simulink model "DFADAS2_SenFus_v1_201204RC_training_210115"  (R2018b)
settings: Solver=FixedStepDiscrete  StartTime=0.0  StopTime=inf  FixedStep=0.002  RelTol=1e-3  EnableMultiTasking=on
PreLoadFcn:
  | RTWConfigurationCB('preloadfcn', bdroot);
libraries: canmsglib x108, simulink x48, canfdmsglib x12
(part 7 of 28)

== system DFADAS2_SenFus_v1_201204RC_training_210115/Signal Input (Input)/Signal Input (10ms) (Input10)/VehInfo/EPS Signal Receive and Processing (EPSRx) ==
  note: Level: 3
  Bus Creator : BusCreator  Inputs=4
  CAN Unpack : canmsglib/CAN Unpack  CANdbFile=F:\LD\3_simulinkModel_13b\TJAHWA\ADAS_D53_PSA1CAN_LiPiao_DLC.dbc  MsgList=EPS_495_PSA1  MsgName=EPS_495_PSA1  MsgIDType=Standard (11-bit identifier)  MsgIdentifier=1173  MsgLength=4  SignalInfo=Power_steering_status$14$2$2$2$1$0$1$0$-Inf$Inf$#State_indicating_steering_or_not$17$1$2$2$1$0$1$0$-Inf$Inf$#State_of_EPS_for_LKA_function$18$3$2$2$1$0$1$0$-Inf$Inf$#Steering_wheel_torque$0$8$2$1$1$0$2.500000e-01$0$-32$3.150000e+01$#Torque_limitation_if_DAE_limit$16$1$2$2$1$0$1$0$-Inf$Inf$#  NSignals=5  IDPort=off  TimestampPort=off  ErrorPort=off  RemotePort=off  LengthPort=off  StatusPort=off  StartBits=str2num('[int32(14);int32(17);int32(18);int32(0);int32(16)]')  SignalSizes=str2num('[int32(2);int32(1);int32(3);int32(8);int32(1)]')  ByteOrders=str2num('[int32(2);int32(2);int32(2);int32(2);int32(2)]')  DataTypes=str2num('[int32(2);int32(2);int32(2);int32(1);int32(2)]')  MultiplexTypes=str2num('[int32(1);int32(1);int32(1);int32(1);int32(1)]')  MultiplexValues=str2num('[double(0);double(0);double(0);double(0);double(0)]')  Factors=str2num('[double(1);double(1);double(1);double(2.500000e-01);double(1)]')  Offsets=str2num('[double(0);double(0);double(0);double(0);double(0)]')  Minimums=str2num('[double(-Inf);double(-Inf);double(-Inf);double(-32);double(-Inf)]')  Maximums=str2num('[double(Inf);double(Inf);double(Inf);double(3.150000e+01);double(Inf)]')  ApplyMinMax=off
      settings: SourceProductName=Simulink Real-Time  SourceProductBaseCode=XP  DataFormat=CANdb specified signals
  Data Type Conversion : DataTypeConversion  OutDataTypeStr=uint16
  Data Type Conversion1 : DataTypeConversion  OutDataTypeStr=single
  Data Type Conversion2 : DataTypeConversion  OutDataTypeStr=uint16
  Data Type Conversion3 : DataTypeConversion  OutDataTypeStr=uint16
  S-Function1 : S-Function  FunctionName=NSTC297CANReceiveBlkLib  Parameters=|  SFunctionDeploymentMode=off  EnableBusSupport=off  mask(NSTC297 CAN Receive){Ns_DeviceID=ADAS Control Unit Gen2, Ns_ChannelNum=4, Ns_FrameID=1173, Ns_IsVirtualFrame=off, Ns_RoleInVirtualFrame=Header Frame, Ns_HeaderFrameID=0, Ns_VirtualFrameStatusFlg=off, Ns_IncompleteFrameCntFlg=off, Ns_OverflowCntFlg=off, Ns_FrameBufferSize=1, Ns_SampleTime=0.01}
      | uint16(Ns_DeviceID),
      | uint16(Ns_ChannelNum),
      | uint32(Ns_FrameID),
      | uint8(Ns_IsVirtualFrame),
      | uint16(Ns_RoleInVirtualFrame),
      | uint32(Ns_HeaderFrameID),
      | uint8(Ns_VirtualFrameStatusFlg),
      | uint8(Ns_IncompleteFrameCntFlg),
      | uint8(Ns_OverflowCntFlg),
      | uint16(Ns_FrameBufferSize),
      | double(Ns_SampleTime)
      mask prompts: Ns_DeviceID "Device:"; Ns_ChannelNum "Channel number:"; Ns_FrameID "Frame ID:"; Ns_IsVirtualFrame "Belong to a virtual frame"; Ns_RoleInVirtualFrame "Position in virtual frame:"; Ns_HeaderFrameID "Header frame ID:"; Ns_VirtualFrameStatusFlg "Current virtural frame status output"; Ns_IncompleteFrameCntFlg "Incomplete virtual frame count output"; Ns_OverflowCntFlg "Overflow count output"; Ns_FrameBufferSize "Frame buffer size:"; Ns_SampleTime "Sample time:"
      mask init:
      | NSTC297CANReceive_callback('portlabels');
      mask TypeOptions Ns_DeviceID: General Control Unit Gen2 | ADAS Control Unit Gen2
      mask TypeOptions Ns_ChannelNum: 0 | 1 | 2 | 3 | 4 | 5
      mask Callback Ns_IsVirtualFrame: NSTC297CANReceive_callback('Belong to a virtual frame');
      mask TypeOptions Ns_RoleInVirtualFrame: Header Frame | Data Frame | Trailer Frame
      mask Callback Ns_RoleInVirtualFrame: NSTC297CANReceive_callback('Position in virtual frame');
      mask Display: color('blue');text(0.02,0.9,'NovSteeds TC297','horizontalAlignment','left');color('blue');text(0.5,0.7,'CAN Receive','horizontalAlignment','center');color('black');text(0.5,0.6,'Channel: 4','horizontalAlignment','center');text(0.5,0.5,'ID: 1173','horizontalAlignment','center');text(0.5,0.4,'Virtual Frame: No','horizontalAlignment','center');port_label('output',1, 'RemainderCnt');port_label('output',2, 'Msg');
  uint16_1 : Constant  Value=0  OutDataTypeStr=uint16
  EPSRx_bsEPSInfo : Outport
  EPSRx_efEPSFaultSyn : Outport  Port=2
  wires:
  Bus Creator/1 -> EPSRx_bsEPSInfo/1
  uint16_1/1 -> EPSRx_efEPSFaultSyn/1
  Data Type Conversion/1 -> Bus Creator/3  "EPSRx_stEPSCtlState"
  Data Type Conversion1/1 -> Bus Creator/4  "EPSRx_trqSWTrq"
  CAN Unpack/1 -> Data Type Conversion2/1
  Data Type Conversion2/1 -> Bus Creator/1  "EPSRx_efEPSErrState"
  S-Function1/2 -> CAN Unpack/1
  CAN Unpack/4 -> Data Type Conversion1/1
  CAN Unpack/3 -> Data Type Conversion/1
  CAN Unpack/2 -> Data Type Conversion3/1
  Data Type Conversion3/1 -> Bus Creator/2  "EPSRx_stHandOff"

== system DFADAS2_SenFus_v1_201204RC_training_210115/Signal Input (Input)/Signal Input (10ms) (Input10)/VehInfo/ForwardVeh_sigback  ==
  Bus Creator : BusCreator  Inputs=3
  CAN Unpack2 : canmsglib/CAN Unpack  CANdbFile=D:\document_ljj\2020_7\ADAS_ECU_PSA1_CAN_V2_v20190520.dbc  MsgList=ADAS_4F7_PSA1  MsgName=SpdDet1_0  MsgIDType=Standard (11-bit identifier)  MsgIdentifier=374  MsgLength=8  SignalInfo=vVeh1Spd$0$16$1$2$1$0$0.01$0$0$300$#lVeh1Dist$16$16$1$1$1$0$1$0$-30000$30000$#aVeh1Acc$32$16$1$1$1$0$0.01$0$-3$3$#  NSignals=3  IDPort=off  TimestampPort=off  ErrorPort=off  RemotePort=off  LengthPort=off  StatusPort=off  StartBits=str2num('[int32(0);int32(16);int32(32)]')  SignalSizes=str2num('[int32(16);int32(16);int32(16)]')  ByteOrders=str2num('[int32(1);int32(1);int32(1)]')  DataTypes=str2num('[int32(2);int32(1);int32(1)]')  MultiplexTypes=str2num('[int32(1);int32(1);int32(1)]')  MultiplexValues=str2num('[double(0);double(0);double(0)]')  Factors=str2num('[double(0.01);double(1);double(0.01)]')  Offsets=str2num('[double(0);double(0);double(0)]')  Minimums=str2num('[double(0);double(-30000);double(-3)]')  Maximums=str2num('[double(300);double(30000);double(3)]')  ApplyMinMax=off
      settings: SourceProductName=Simulink Real-Time  SourceProductBaseCode=XP
  Constant : Constant  Value=80
  Constant1 : Constant  Value=30000
  Constant2 : Constant  Value=0
  S-Function11 : S-Function  FunctionName=NSTC297CANReceiveBlkLib  Parameters=|  SFunctionDeploymentMode=off  EnableBusSupport=off  mask(NSTC297 CAN Receive){Ns_DeviceID=ADAS Control Unit Gen2, Ns_ChannelNum=5, Ns_FrameID=374, Ns_IsVirtualFrame=off, Ns_RoleInVirtualFrame=Header Frame, Ns_HeaderFrameID=0, Ns_VirtualFrameStatusFlg=off, Ns_IncompleteFrameCntFlg=off, Ns_OverflowCntFlg=off, Ns_FrameBufferSize=1, Ns_SampleTime=0.01}
      | uint16(Ns_DeviceID),
      | uint16(Ns_ChannelNum),
      | uint32(Ns_FrameID),
      | uint8(Ns_IsVirtualFrame),
      | uint16(Ns_RoleInVirtualFrame),
      | uint32(Ns_HeaderFrameID),
      | uint8(Ns_VirtualFrameStatusFlg),
      | uint8(Ns_IncompleteFrameCntFlg),
      | uint8(Ns_OverflowCntFlg),
      | uint16(Ns_FrameBufferSize),
      | double(Ns_SampleTime)
      mask prompts: Ns_DeviceID "Device:"; Ns_ChannelNum "Channel number:"; Ns_FrameID "Frame ID:"; Ns_IsVirtualFrame "Belong to a virtual frame"; Ns_RoleInVirtualFrame "Position in virtual frame:"; Ns_HeaderFrameID "Header frame ID:"; Ns_VirtualFrameStatusFlg "Current virtural frame status output"; Ns_IncompleteFrameCntFlg "Incomplete virtual frame count output"; Ns_OverflowCntFlg "Overflow count output"; Ns_FrameBufferSize "Frame buffer size:"; Ns_SampleTime "Sample time:"
      mask init:
      | NSTC297CANReceive_callback('portlabels');
      mask TypeOptions Ns_DeviceID: General Control Unit Gen2 | ADAS Control Unit Gen2
      mask TypeOptions Ns_ChannelNum: 0 | 1 | 2 | 3 | 4 | 5
      mask Callback Ns_IsVirtualFrame: NSTC297CANReceive_callback('Belong to a virtual frame');
      mask TypeOptions Ns_RoleInVirtualFrame: Header Frame | Data Frame | Trailer Frame
      mask Callback Ns_RoleInVirtualFrame: NSTC297CANReceive_callback('Position in virtual frame');
      mask Display: color('blue');text(0.02,0.9,'NovSteeds TC297','horizontalAlignment','left');color('blue');text(0.5,0.7,'CAN Receive','horizontalAlignment','center');color('black');text(0.5,0.6,'Channel: 5','horizontalAlignment','center');text(0.5,0.5,'ID: 374','horizontalAlignment','center');text(0.5,0.4,'Virtual Frame: No','horizontalAlignment','center');port_label('output',1, 'RemainderCnt');port_label('output',2, 'Msg');
  SpdReq_bsSpdDet1info : Outport
  wires:
  S-Function11/2 -> CAN Unpack2/1
  Constant/1 -> Bus Creator/1  "SpdDet1_vVeh1Spd"
  Constant1/1 -> Bus Creator/2  "SpdDet1_lVeh1Dist"
  Constant2/1 -> Bus Creator/3  "SpdDet1_aVeh1Acc"
  Bus Creator/1 -> SpdReq_bsSpdDet1info/1

== system DFADAS2_SenFus_v1_201204RC_training_210115/Signal Input (Input)/Signal Input (10ms) (Input10)/VehInfo/From ACC (From ACC) ==
  CAN Unpack3 : canmsglib/CAN Unpack  CANdbFile=F:\LD\1_simulinkModel_10b\TJAHWA\CAN0_VehicleAllSignalWhAdd_LC.dbc  MsgList=(none)  MsgName=ACC2TJA  MsgIDType=Standard (11-bit identifier)  MsgIdentifier=665  MsgLength=8  SignalInfo=ACC_SMState$8$8$2$2$1$0$1$0$0$255$#CheckSum$56$8$2$2$1$0$1$0$0$255$#RollingCounter$0$8$2$2$1$0$1$0$0$255$#  NSignals=3  IDPort=off  TimestampPort=off  ErrorPort=off  RemotePort=off  LengthPort=off  StatusPort=off  StartBits=str2num('[int32(8);int32(56);int32(0)]')  SignalSizes=str2num('[int32(8);int32(8);int32(8)]')  ByteOrders=str2num('[int32(2);int32(2);int32(2)]')  DataTypes=str2num('[int32(2);int32(2);int32(2)]')  MultiplexTypes=str2num('[int32(1);int32(1);int32(1)]')  MultiplexValues=str2num('[double(0);double(0);double(0)]')  Factors=str2num('[double(1);double(1);double(1)]')  Offsets=str2num('[double(0);double(0);double(0)]')  Minimums=str2num('[double(0);double(0);double(0)]')  Maximums=str2num('[double(255);double(255);double(255)]')  ApplyMinMax=off
      settings: SourceProductName=Simulink Real-Time  SourceProductBaseCode=XP
  Data Type Conversion : DataTypeConversion  OutDataTypeStr=uint16
  S-Function1 : S-Function  FunctionName=NSTC297CANReceiveBlkLib  Parameters=|  SFunctionDeploymentMode=off  EnableBusSupport=off  mask(NSTC297 CAN Receive){Ns_DeviceID=ADAS Control Unit Gen2, Ns_ChannelNum=4, Ns_FrameID=665, Ns_IsVirtualFrame=off, Ns_RoleInVirtualFrame=Header Frame, Ns_HeaderFrameID=0, Ns_VirtualFrameStatusFlg=off, Ns_IncompleteFrameCntFlg=off, Ns_OverflowCntFlg=off, Ns_FrameBufferSize=1, Ns_SampleTime=0.01}
      | uint16(Ns_DeviceID),
      | uint16(Ns_ChannelNum),
      | uint32(Ns_FrameID),
      | uint8(Ns_IsVirtualFrame),
      | uint16(Ns_RoleInVirtualFrame),
      | uint32(Ns_HeaderFrameID),
      | uint8(Ns_VirtualFrameStatusFlg),
      | uint8(Ns_IncompleteFrameCntFlg),
      | uint8(Ns_OverflowCntFlg),
      | uint16(Ns_FrameBufferSize),
      | double(Ns_SampleTime)
      mask prompts: Ns_DeviceID "Device:"; Ns_ChannelNum "Channel number:"; Ns_FrameID "Frame ID:"; Ns_IsVirtualFrame "Belong to a virtual frame"; Ns_RoleInVirtualFrame "Position in virtual frame:"; Ns_HeaderFrameID "Header frame ID:"; Ns_VirtualFrameStatusFlg "Current virtural frame status output"; Ns_IncompleteFrameCntFlg "Incomplete virtual frame count output"; Ns_OverflowCntFlg "Overflow count output"; Ns_FrameBufferSize "Frame buffer size:"; Ns_SampleTime "Sample time:"
      mask init:
      | NSTC297CANReceive_callback('portlabels');
      mask TypeOptions Ns_DeviceID: General Control Unit Gen2 | ADAS Control Unit Gen2
      mask TypeOptions Ns_ChannelNum: 0 | 1 | 2 | 3 | 4 | 5
      mask Callback Ns_IsVirtualFrame: NSTC297CANReceive_callback('Belong to a virtual frame');
      mask TypeOptions Ns_RoleInVirtualFrame: Header Frame | Data Frame | Trailer Frame
      mask Callback Ns_RoleInVirtualFrame: NSTC297CANReceive_callback('Position in virtual frame');
      mask Display: color('blue');text(0.02,0.9,'NovSteeds TC297','horizontalAlignment','left');color('blue');text(0.5,0.7,'CAN Receive','horizontalAlignment','center');color('black');text(0.5,0.6,'Channel: 4','horizontalAlignment','center');text(0.5,0.5,'ID: 665','horizontalAlignment','center');text(0.5,0.4,'Virtual Frame: No','horizontalAlignment','center');port_label('output',1, 'RemainderCnt');port_label('output',2, 'Msg');
  From ACC_stACCState : Outport
  From ACC_efFromACCFaultSyn : Outport  Port=2
  From_ACC_stACCState_Mon : Outport  Port=3
  wires:
  S-Function1/2 -> CAN Unpack3/1
  Data Type Conversion/1 -> From ACC_stACCState/1
  CAN Unpack3/1 -> From_ACC_stACCState_Mon/1, Data Type Conversion/1

== system DFADAS2_SenFus_v1_201204RC_training_210115/Signal Input (Input)/Signal Input (10ms) (Input10)/VehInfo/Function Keys State Receive and Processing (FKeyStRx) ==
  Fault Synthesis (FaultSyn) : Subsystem
  Key Enable CAN Frame PreProcess (KeyEnaCANFrmPPrcs) : Subsystem
  FKeyStRx_stFKeyState : Outport
  FKeyStRx_efFKeyFaultSyn : Outport  Port=2
  wires:
  Fault Synthesis (FaultSyn)/1(FaultSyn_efFaultSyn) -> FKeyStRx_efFKeyFaultSyn/1
  Key Enable CAN Frame PreProcess (KeyEnaCANFrmPPrcs)/1(IC_RightSteeringWheelSwitchSig) -> FKeyStRx_stFKeyState/1

== system DFADAS2_SenFus_v1_201204RC_training_210115/Signal Input (Input)/Signal Input (10ms) (Input10)/VehInfo/MP5 Signal Receive (MP5Rx)1 ==
  note: Level: 3, [1.1.2]
  Bus Creator : BusCreator  Inputs=2
  CAN Diagnosis (CANDia) : Subsystem  Commented=on
  CAN Receive Sample Time : Constant  Value=0.02  OutDataTypeStr=single  SampleTime=-1
  CAN Unpack1 : canmsglib/CAN Unpack  CANdbFile=F:\LD\3_simulinkModel_13b\TJAHWA\ADAS_D53_PSA1CAN_LiPiao_DLC.dbc  MsgList=GW_550_PSA1  MsgName=GW_550_PSA1  MsgIDType=Standard (11-bit identifier)  MsgIdentifier=1360  MsgLength=8  SignalInfo=GW_Mp5_ISA_Switch$3$2$2$2$1$0$1$0$0$3$#GW_Mp5_TSR_Switch$1$2$2$2$1$0$1$0$0$3$#LC_Mode$6$2$2$2$1$0$1$0$0$3$#LKA_main_switch$5$1$2$2$1$0$1$0$0$1$#  NSignals=4  IDPort=off  TimestampPort=off  ErrorPort=off  RemotePort=off  LengthPort=off  StatusPort=off  StartBits=str2num('[int32(3);int32(1);int32(6);int32(5)]')  SignalSizes=str2num('[int32(2);int32(2);int32(2);int32(1)]')  ByteOrders=str2num('[int32(2);int32(2);int32(2);int32(2)]')  DataTypes=str2num('[int32(2);int32(2);int32(2);int32(2)]')  MultiplexTypes=str2num('[int32(1);int32(1);int32(1);int32(1)]')  MultiplexValues=str2num('[double(0);double(0);double(0);double(0)]')  Factors=str2num('[double(1);double(1);double(1);double(1)]')  Offsets=str2num('[double(0);double(0);double(0);double(0)]')  Minimums=str2num('[double(0);double(0);double(0);double(0)]')  Maximums=str2num('[double(3);double(3);double(3);double(1)]')  ApplyMinMax=off
      settings: SourceProductName=Simulink Real-Time  SourceProductBaseCode=XP  DataFormat=CANdb specified signals
  Data Type Conversion : DataTypeConversion  OutDataTypeStr=uint16
  Data Type Conversion1 : DataTypeConversion  OutDataTypeStr=uint16
  Rate Transition : RateTransition  Deterministic=off  OutPortSampleTime=0.01
  Rate Transition1 : RateTransition  Deterministic=off  OutPortSampleTime=0.01
  S-Function1 : S-Function  FunctionName=NSTC297CANReceiveBlkLib  Parameters=|  SFunctionDeploymentMode=off  EnableBusSupport=off  mask(NSTC297 CAN Receive){Ns_DeviceID=ADAS Control Unit Gen2, Ns_ChannelNum=4, Ns_FrameID=1360, Ns_IsVirtualFrame=off, Ns_RoleInVirtualFrame=Header Frame, Ns_HeaderFrameID=0, Ns_VirtualFrameStatusFlg=off, Ns_IncompleteFrameCntFlg=off, Ns_OverflowCntFlg=off, Ns_FrameBufferSize=1, Ns_SampleTime=0.5}
      | uint16(Ns_DeviceID),
      | uint16(Ns_ChannelNum),
      | uint32(Ns_FrameID),
      | uint8(Ns_IsVirtualFrame),
      | uint16(Ns_RoleInVirtualFrame),
      | uint32(Ns_HeaderFrameID),
      | uint8(Ns_VirtualFrameStatusFlg),
      | uint8(Ns_IncompleteFrameCntFlg),
      | uint8(Ns_OverflowCntFlg),
      | uint16(Ns_FrameBufferSize),
      | double(Ns_SampleTime)
      mask prompts: Ns_DeviceID "Device:"; Ns_ChannelNum "Channel number:"; Ns_FrameID "Frame ID:"; Ns_IsVirtualFrame "Belong to a virtual frame"; Ns_RoleInVirtualFrame "Position in virtual frame:"; Ns_HeaderFrameID "Header frame ID:"; Ns_VirtualFrameStatusFlg "Current virtural frame status output"; Ns_IncompleteFrameCntFlg "Incomplete virtual frame count output"; Ns_OverflowCntFlg "Overflow count output"; Ns_FrameBufferSize "Frame buffer size:"; Ns_SampleTime "Sample time:"
      mask init:
      | NSTC297CANReceive_callback('portlabels');
      mask TypeOptions Ns_DeviceID: General Control Unit Gen2 | ADAS Control Unit Gen2
      mask TypeOptions Ns_ChannelNum: 0 | 1 | 2 | 3 | 4 | 5
      mask Callback Ns_IsVirtualFrame: NSTC297CANReceive_callback('Belong to a virtual frame');
      mask TypeOptions Ns_RoleInVirtualFrame: Header Frame | Data Frame | Trailer Frame
      mask Callback Ns_RoleInVirtualFrame: NSTC297CANReceive_callback('Position in virtual frame');
      mask Display: color('blue');text(0.02,0.9,'NovSteeds TC297','horizontalAlignment','left');color('blue');text(0.5,0.7,'CAN Receive','horizontalAlignment','center');color('black');text(0.5,0.6,'Channel: 4','horizontalAlignment','center');text(0.5,0.5,'ID: 1360','horizontalAlignment','center');text(0.5,0.4,'Virtual Frame: No','horizontalAlignment','center');port_label('output',1, 'RemainderCnt');port_label('output',2, 'Msg');
  Time Limit : Constant  OutDataTypeStr=single  SampleTime=-1
  MP5Rx_bsMP5Info : Outport
  wires:
  Rate Transition/1 -> Data Type Conversion/1
  S-Function1/2 -> CAN Diagnosis (CANDia)/4(CANDia_regCANMsg), CAN Unpack1/1
  CAN Receive Sample Time/1 -> CAN Diagnosis (CANDia)/1(CANDia_tiCANRxSmplT)
  Time Limit/1 -> CAN Diagnosis (CANDia)/2(CANDia_tiTLim)
  S-Function1/1 -> CAN Diagnosis (CANDia)/3(CANDia_cfNewFlg)
  Rate Transition1/1 -> Data Type Conversion1/1
  Data Type Conversion/1 -> Bus Creator/1  "Mp5_LaneKeepingActivation"
  Data Type Conversion1/1 -> Bus Creator/2  "Mp5_LaneKeepingModeRequest"
  Bus Creator/1 -> MP5Rx_bsMP5Info/1
  CAN Unpack1/4 -> Rate Transition/1
  CAN Unpack1/3 -> Rate Transition1/1

== system DFADAS2_SenFus_v1_201204RC_training_210115/Signal Input (Input)/Signal Input (10ms) (Input10)/VehInfo/Powertrain State Receive and Processing (PTRx) ==
  Bus Creator1 : BusCreator  Inputs=2
  Bus Creator2 : BusCreator  Inputs=2
  EMS State Receive and Processing (EMSRx) : Subsystem
  TCU State Receive and Processing (TCURx) : Subsystem
  PTRx_bsPTState : Outport
  PTRx_bsPTFaultSyn : Outport  Port=2
  wires:
  Bus Creator2/1 -> PTRx_bsPTFaultSyn/1
  Bus Creator1/1 -> PTRx_bsPTState/1
  EMS State Receive and Processing (EMSRx)/1(EMSRx_bsEMSState) -> Bus Creator1/1  "EMSRx_bsEMSState"
  EMS State Receive and Processing (EMSRx)/2(EMSRx_bsEMSFaultSyn) -> Bus Creator2/1
  TCU State Receive and Processing (TCURx)/1(TCURx_bsTCUState) -> Bus Creator1/2  "TCURx_bsTCUState"
  TCU State Receive and Processing (TCURx)/2(TCURx_bsTCUFaultSyn) -> Bus Creator2/2

== system DFADAS2_SenFus_v1_201204RC_training_210115/Signal Input (Input)/Signal Input (10ms) (Input10)/VehInfo/Steeing Wheel Angle Receive and Processing (SWARx) ==
  Bus Creator1 : BusCreator  Inputs=4
  Bus Creator2 : BusCreator  Inputs=2
  CAN Unpack : canmsglib/CAN Unpack  CANdbFile=F:\LD\3_simulinkModel_13b\TJAHWA\ADAS_D53_PSA1CAN_LiPiao_DLC.dbc  MsgList=EPS_305_PSA1  MsgName=EPS_305_PSA1  MsgIDType=Standard (11-bit identifier)  MsgIdentifier=773  MsgLength=7  SignalInfo=Absolute_Steering_Wheel_angle$54$1$2$2$1$0$1$0$-Inf$Inf$#Initialization_steering_angle$55$1$2$2$1$0$1$0$-Inf$Inf$#Internal_SWS_status$24$1$2$2$1$0$1$0$-Inf$Inf$#SWS_calibration$25$1$2$2$1$0$1$0$-Inf$Inf$#SWS_checksum$36$4$2$2$1$0$1$0$-Inf$Inf$#SWS_fault_code$27$4$2$2$1$0$1$0$-Inf$Inf$#SWS_trim$26$1$2$2$1$0$1$0$-Inf$Inf$#Steering_wheel_angle$8$16$2$1$1$0$1.000000e-01$0$-780$780$#Steering_wheel_rotation_speed$16$8$2$2$1$0$4$0$0$1016$#Steering_wheel_sensor_direction$31$1$2$2$1$0$1$0$-Inf$Inf$#bits_Compute_counter_for_SWS$32$4$2$2$1$0$1$0$0$15$#indication_of_steering_wheel$52$2$2$2$1$0$1$0$-Inf$Inf$#  NSignals=12  IDPort=off  TimestampPort=off  ErrorPort=off  RemotePort=off  LengthPort=off  StatusPort=off  StartBits=str2num('[int32(54);int32(55);int32(24);int32(25);int32(36);int32(27);int32(26);int32(8);int32(16);int32(31);int32(32);int32(52)]')  SignalSizes=str2num('[int32(1);int32(1);int32(1);int32(1);int32(4);int32(4);int32(1);int32(16);int32(8);int32(1);int32(4);int32(2)]')  ByteOrders=str2num('[int32(2);int32(2);int32(2);int32(2);int32(2);int32(2);int32(2);int32(2);int32(2);int32(2);int32(2);int32(2)]')  DataTypes=str2num('[int32(2);int32(2);int32(2);int32(2);int32(2);int32(2);int32(2);int32(1);int32(2);int32(2);int32(2);int32(2)]')  MultiplexTypes=str2num('[int32(1);int32(1);int32(1);int32(1);int32(1);int32(1);int32(1);int32(1);int32(1);int32(1);int32(1);int32(1)]')  MultiplexValues=str2num('[double(0);double(0);double(0);double(0);double(0);double(0);double(0);double(0);double(0);double(0);double(0);double(0)]')  Factors=str2num('[double(1);double(1);double(1);double(1);double(1);double(1);double(1);double(1.000000e-01);double(4);double(1);double(1);double(1)]')  Offsets=str2num('[double(0);double(0);double(0);double(0);double(0);double(0);double(0);double(0);double(0);double(0);double(0);double(0)]')  Minimums=str2num('[double(-Inf);double(-Inf);double(-Inf);double(-Inf);double(-Inf);double(-Inf);double(-Inf);double(-780);double(0);double(-Inf);double(0);double(-Inf)]')  Maximums=str2num('[double(Inf);double(Inf);double(Inf);double(Inf);double(Inf);double(Inf);double(Inf);double(780);double(1016);double(Inf);double(15);double(Inf)]')  ApplyMinMax=off
      settings: SourceProductName=Simulink Real-Time  SourceProductBaseCode=XP  DataFormat=CANdb specified signals
  Data Type Conversion46 : DataTypeConversion  OutDataTypeStr=uint16
  Data Type Conversion47 : DataTypeConversion  OutDataTypeStr=uint16
  S-Function1 : S-Function  FunctionName=NSTC297CANReceiveBlkLib  Parameters=|  SFunctionDeploymentMode=off  EnableBusSupport=off  mask(NSTC297 CAN Receive){Ns_DeviceID=ADAS Control Unit Gen2, Ns_ChannelNum=4, Ns_FrameID=773, Ns_IsVirtualFrame=off, Ns_RoleInVirtualFrame=Header Frame, Ns_HeaderFrameID=0, Ns_VirtualFrameStatusFlg=off, Ns_IncompleteFrameCntFlg=off, Ns_OverflowCntFlg=off, Ns_FrameBufferSize=1, Ns_SampleTime=0.01}
      | uint16(Ns_DeviceID),
      | uint16(Ns_ChannelNum),
      | uint32(Ns_FrameID),
      | uint8(Ns_IsVirtualFrame),
      | uint16(Ns_RoleInVirtualFrame),
      | uint32(Ns_HeaderFrameID),
      | uint8(Ns_VirtualFrameStatusFlg),
      | uint8(Ns_IncompleteFrameCntFlg),
      | uint8(Ns_OverflowCntFlg),
      | uint16(Ns_FrameBufferSize),
      | double(Ns_SampleTime)
      mask prompts: Ns_DeviceID "Device:"; Ns_ChannelNum "Channel number:"; Ns_FrameID "Frame ID:"; Ns_IsVirtualFrame "Belong to a virtual frame"; Ns_RoleInVirtualFrame "Position in virtual frame:"; Ns_HeaderFrameID "Header frame ID:"; Ns_VirtualFrameStatusFlg "Current virtural frame status output"; Ns_IncompleteFrameCntFlg "Incomplete virtual frame count output"; Ns_OverflowCntFlg "Overflow count output"; Ns_FrameBufferSize "Frame buffer size:"; Ns_SampleTime "Sample time:"
      mask init:
      | NSTC297CANReceive_callback('portlabels');
      mask TypeOptions Ns_DeviceID: General Control Unit Gen2 | ADAS Control Unit Gen2
      mask TypeOptions Ns_ChannelNum: 0 | 1 | 2 | 3 | 4 | 5
      mask Callback Ns_IsVirtualFrame: NSTC297CANReceive_callback('Belong to a virtual frame');
      mask TypeOptions Ns_RoleInVirtualFrame: Header Frame | Data Frame | Trailer Frame
      mask Callback Ns_RoleInVirtualFrame: NSTC297CANReceive_callback('Position in virtual frame');
      mask Display: color('blue');text(0.02,0.9,'NovSteeds TC297','horizontalAlignment','left');color('blue');text(0.5,0.7,'CAN Receive','horizontalAlignment','center');color('black');text(0.5,0.6,'Channel: 4','horizontalAlignment','center');text(0.5,0.5,'ID: 773','horizontalAlignment','center');text(0.5,0.4,'Virtual Frame: No','horizontalAlignment','center');port_label('output',1, 'RemainderCnt');port_label('output',2, 'Msg');
  uint16_1 : Constant  Value=0  OutDataTypeStr=uint16
  uint16_2 : Constant  Value=0  OutDataTypeStr=uint16
  SWARx_bsSWAInfo : Outport
  SWARx_bsSWAFaultSyn : Outport  Port=2
  wires:
  S-Function1/2 -> CAN Unpack/1
  CAN Unpack/8 -> Bus Creator1/1  "SWARx_phiSWA"
  CAN Unpack/9 -> Bus Creator1/2  "SWARx_dphiSWARotSpd"
  Bus Creator1/1 -> SWARx_bsSWAInfo/1
  Bus Creator2/1 -> SWARx_bsSWAFaultSyn/1
  uint16_1/1 -> Bus Creator2/1
  uint16_2/1 -> Bus Creator2/2
  Data Type Conversion47/1 -> Bus Creator1/3  "Internal_SWS_status"
  Data Type Conversion46/1 -> Bus Creator1/4  "SWS_fault_code"
  CAN Unpack/6 -> Data Type Conversion46/1
  CAN Unpack/3 -> Data Type Conversion47/1

== system DFADAS2_SenFus_v1_201204RC_training_210115/Signal Input (Input)/Signal Input (10ms) (Input10)/VehInfo/Vehicle Movement Signal Receive and Processing (VehMovRx) ==
  Bus Creator1 : BusCreator  Inputs=12
  Bus Creator2 : BusCreator  Inputs=4
  Fault Synthesis (FaultSyn) : Subsystem
  Fault Synthesis (FaultSyn)1 : Subsystem
  Fault Synthesis (FaultSyn)2 : Subsystem
  VehLonAcc CAN Frame PreProcess (VehLonAccCANFrmPPrcs) : Subsystem
  VehSpd CAN Frame PreProcess (VehSpdCANFrmPPrcs) : Subsystem
  Yaw State CAN Frame PreProcess (YawCANFrmPPrcs) : Subsystem
  uint16_1 : Constant  Value=0  OutDataTypeStr=uint16
  VehMovRx_bsVehMovInfo : Outport
  VehMovRx_efVehMovFaultSyn : Outport  Port=2
  wires:
  Fault Synthesis (FaultSyn)1/1(FaultSyn_efFaultSyn) -> Fault Synthesis (FaultSyn)2/2(in2)
  Fault Synthesis (FaultSyn)/1(FaultSyn_efFaultSyn) -> Fault Synthesis (FaultSyn)2/1(in1)
  Fault Synthesis (FaultSyn)2/1(FaultSyn_efFaultSyn) -> Bus Creator2/1
  VehSpd CAN Frame PreProcess (VehSpdCANFrmPPrcs)/7(Out7) -> Fault Synthesis (FaultSyn)1/7(in7)
  VehSpd CAN Frame PreProcess (VehSpdCANFrmPPrcs)/6(Out6) -> Fault Synthesis (FaultSyn)1/6(in6)
  VehSpd CAN Frame PreProcess (VehSpdCANFrmPPrcs)/5(CANFrmPPrcs_vVehSpd) -> Bus Creator1/3, Fault Synthesis (FaultSyn)1/5(in5)  "VehMovRx_vVehSpd"
  VehSpd CAN Frame PreProcess (VehSpdCANFrmPPrcs)/4(Vehiclespeed_unavailability_flag) -> Bus Creator1/11, Fault Synthesis (FaultSyn)1/4(in4)  "Vehiclespeed_unavailability_flag"
  VehSpd CAN Frame PreProcess (VehSpdCANFrmPPrcs)/3(out) -> Fault Synthesis (FaultSyn)1/3(in3), Bus Creator1/5  "ESC_BrakeOilPress"
  VehSpd CAN Frame PreProcess (VehSpdCANFrmPPrcs)/2(Vehicle_driving_direction) -> Bus Creator1/10, Fault Synthesis (FaultSyn)1/2(in2)  "Vehicle_driving_direction"
  VehSpd CAN Frame PreProcess (VehSpdCANFrmPPrcs)/1(Out1) -> Fault Synthesis (FaultSyn)1/1(in1)
  Yaw State CAN Frame PreProcess (YawCANFrmPPrcs)/5(Out5) -> Fault Synthesis (FaultSyn)/5(in5)
  Yaw State CAN Frame PreProcess (YawCANFrmPPrcs)/4(Out4) -> Fault Synthesis (FaultSyn)/4(in4)
  Yaw State CAN Frame PreProcess (YawCANFrmPPrcs)/2(Brake_pedal_disabled_UC_Brake) -> Fault Synthesis (FaultSyn)/2(in2), Bus Creator1/12  "Brake_pedal_disabled_UC_Brake"
  Yaw State CAN Frame PreProcess (YawCANFrmPPrcs)/1(YawCANFrmPPrcs_aLAcc) -> Bus Creator1/1, Fault Synthesis (FaultSyn)/1(in1)  "VehMovRx_aLAcc"
  Yaw State CAN Frame PreProcess (YawCANFrmPPrcs)/3(YawCANFrmPPrcs_arYR) -> Bus Creator1/2, Fault Synthesis (FaultSyn)/3(in3)  "VehMovRx_dphiYawRate"
  Bus Creator1/1 -> VehMovRx_bsVehMovInfo/1
  Bus Creator2/1 -> VehMovRx_efVehMovFaultSyn/1
  uint16_1/1 -> Bus Creator2/4, Bus Creator2/3, Bus Creator2/2
  VehLonAcc CAN Frame PreProcess (VehLonAccCANFrmPPrcs)/1(ESC_LongitudinalAcc) -> Bus Creator1/4  "ESC_LongitudinalAcc"
  VehLonAcc CAN Frame PreProcess (VehLonAccCANFrmPPrcs)/2(ESC_ACC_Status) -> Bus Creator1/6  "ESC_ACC_Status"
  VehLonAcc CAN Frame PreProcess (VehLonAccCANFrmPPrcs)/3(ESC_AEB_Status) -> Bus Creator1/7  "ESC_AEB_Status"
  VehLonAcc CAN Frame PreProcess (VehLonAccCANFrmPPrcs)/4(Message_from_ESC_informing) -> Bus Creator1/8  "Message_from_ESC_informing"
  VehLonAcc CAN Frame PreProcess (VehLonAccCANFrmPPrcs)/5(Vehicle_detected_as_stationary) -> Bus Creator1/9  "Vehicle_detected_as_stationary"
